simulink model "fast"  (R2019b)
settings: Solver=FixedStepDiscrete  StartTime=0.0  StopTime=25  FixedStep=Ts_proc  RelTol=1e-3
model workspace: external: MAT-File (data not in the file)
values from neighbouring files (symbols this model uses):
  bma = bm + ba    (= 0.0174)    [datasheet.m]
  bp = 0.0024    [datasheet.m]
  CCR_max = 5250    [datasheet.m]
  eta_g = 0.9    [datasheet.m]
  g = 9.81    [datasheet.m]
  J0 = Jm_eq + Jarm + mp*Larm^2    (= 0.0104704670992)    [datasheet.m]
  Jp = Jp_cm + mp*lp^2    (= 0.004290672)    [datasheet.m]
  Ke = 7.68e-3    (= 0.00768)    [datasheet.m]
  Kg = 70    [datasheet.m]
  Kt = 7.68e-3    (= 0.00768)    [datasheet.m]
  Larm = 0.216    [datasheet.m]
  Lm = 0.18*1e-3    (= 0.00018)    [datasheet.m]
  Lp = 0.337    [datasheet.m]
  lp = 0.156    [datasheet.m]
  mp = 0.127    [datasheet.m]
  Rm = 2.6    [datasheet.m]
  Ts_proc = 1e-3    (= 0.001)    [codegen_init.m]
  volt_max = 6    [datasheet.m]
undefined symbols (not defined in the file or in its folder): DiscIntNeverNeededParam, state_pc_init
settings Model: OrderedModelArguments=off  Creator=Simone  LastModifiedBy=Simone
settings OptimizationCC: DefaultParameterBehavior=Inlined  GainParamInheritBuiltInType=on  UseFloatMulNetSlope=on  UseSpecifiedMinMax=on  InlineInvariantSignals=on  PassReuseOutputArgsAs=Individual arguments  ZeroExternalMemoryAtStartup=off  ZeroInternalMemoryAtStartup=off  NoFixptDivByZeroProtection=on  EfficientFloat2IntCast=on  LifeSpan=1  OptimizeBlockOrder=speed  EfficientTunableParamExpr=on
settings DebuggingCC: SignalInfNanChecking=error  ParameterPrecisionLossMsg=error  ParameterTunabilityLossMsg=error
settings HardwareCC: ProdBitPerLong=64  ProdLongLongMode=on  ProdHWDeviceType=Intel->x86-64 (Linux 64)
settings SFSimCC: MATLABDynamicMemAlloc=off
settings RTWCC: SystemTargetFile=ert.tlc  GenCodeOnly=on  PackageGeneratedCodeAndArtifacts=on  TemplateMakefile=ert_default_tmf  GenerateReport=on  Toolchain=GNU gcc/g++ | gmake (64-bit Linux)  BuildConfiguration=Faster Runs  IncludeHyperlinkInReport=on  LaunchReport=on  GenerateTraceInfo=on  GenerateTraceReport=on  GenerateTraceReportSl=on  GenerateTraceReportSf=on  GenerateTraceReportEml=on  CheckMdlBeforeBuild=Error
settings CodeAppCC: ForceParamTrailComments=on  IgnoreCustomStorageClasses=off  OperatorAnnotations=on  SimulinkDataObjDesc=on  SFDataObjDesc=on  MATLABFcnDesc=on  InsertBlockDesc=on  StateflowObjectComments=on  MATLABSourceComments=on  EnableCustomComments=on  ReqsInCode=on
settings ERTTargetCC: TargetLangStandard=C99 (ISO)  UtilityFuncGeneration=Shared location  CombineSignalStateStructs=on  SuppressErrorStatus=on  SupportAbsoluteTime=off  SupportNonFinite=off  SupportComplex=off  InlinedParameterPlacement=NonHierarchical  ERTCustomFileTemplate=example_file_process.tlc

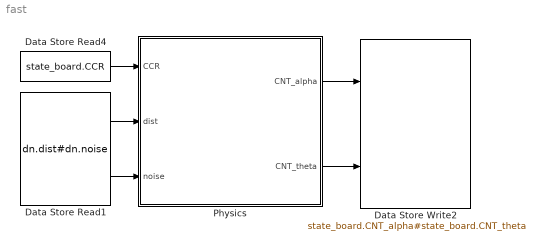
== system fast ==
  Data Store Read1 : DataStoreRead  DataStoreName=dn  DataStoreElements=dn.dist#dn.noise
  Data Store Read4 : DataStoreRead  DataStoreName=state_board  DataStoreElements=state_board.CCR
  Data Store Write2 : DataStoreWrite  DataStoreName=state_board  DataStoreElements=state_board.CNT_alpha#state_board.CNT_theta
  Physics : Subsystem  TreatAsAtomicUnit=on  RTWFcnName=physics  RTWFileName=physics
      settings: RTWSystemCode=Nonreusable function  RTWFcnNameOpts=User specified  RTWFileNameOpts=User specified  FunctionInterfaceSpec=Allow arguments
  wires:
  Data Store Read4/1 -> Physics/1(CCR)
  Physics/1(CNT_alpha) -> Data Store Write2/1
  Physics/2(CNT_theta) -> Data Store Write2/2
  Data Store Read1/1 -> Physics/2(dist)
  Data Store Read1/2 -> Physics/3(noise)

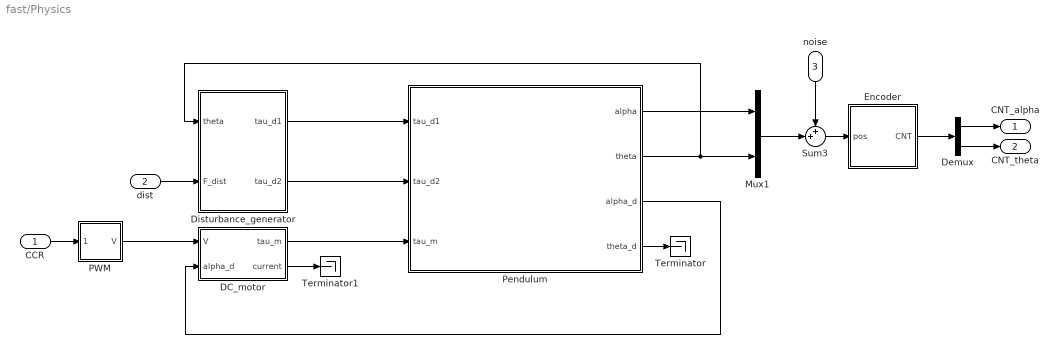
== system fast/Physics ==
  CCR : Inport
  dist : Inport  Port=2
  noise : Inport  Port=3
  DC_motor : Subsystem
  Demux : Demux  Outputs=2
  Disturbance_generator : Subsystem
  Encoder : Subsystem
  Mux1 : Mux  Inputs=2
  PWM : Subsystem
  Pendulum : Subsystem
  Sum3 : Sum  Inputs=++|
  Terminator : Terminator
  Terminator1 : Terminator
  CNT_alpha : Outport
  CNT_theta : Outport  Port=2
  wires:
  Demux/1 -> CNT_alpha/1
  Demux/2 -> CNT_theta/1
  Encoder/1(CNT) -> Demux/1
  Pendulum/4(theta_d) -> Terminator/1
  Mux1/1 -> Sum3/2
  dist/1 -> Disturbance_generator/2(F_dist)
  CCR/1 -> PWM/1(CCR)
  DC_motor/1(tau_m) -> Pendulum/3(tau_m)
  Disturbance_generator/2(tau_d2) -> Pendulum/2(tau_d2)
  Disturbance_generator/1(tau_d1) -> Pendulum/1(tau_d1)
  noise/1 -> Sum3/1
  Sum3/1 -> Encoder/1(pos)
  Pendulum/1(alpha) -> Mux1/1
  Pendulum/2(theta) -> Disturbance_generator/1(theta), Mux1/2
  DC_motor/2(current) -> Terminator1/1
  Pendulum/3(alpha_d) -> DC_motor/2(alpha_d)
  PWM/1(V) -> DC_motor/1(V)

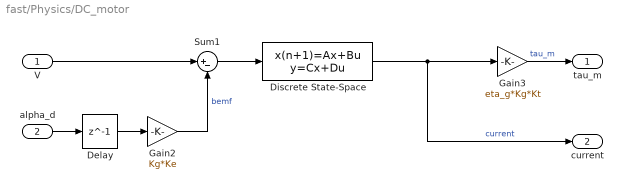
== system fast/Physics/DC_motor ==
  V : Inport
  alpha_d : Inport  Port=2
  Delay : Delay  DelayLength=1  InitialCondition=0
  Discrete State-Space : DiscreteStateSpace  A=-(Rm*Ts_proc - 2*Lm)/(Rm*Ts_proc + 2*Lm)  B=Ts_proc/(2*Lm + Rm*Ts_proc)*(1-(Rm*Ts_proc - 2*Lm)/(Rm*Ts_proc + 2*Lm))  D=Ts_proc/(2*Lm + Rm*Ts_proc)  InitialCondition=single(0)  SampleTime=Ts_proc
  Gain2 : Gain  Gain=Kg*Ke
  Gain3 : Gain  Gain=eta_g*Kg*Kt
  Sum1 : Sum  Inputs=|+-
  tau_m : Outport
  current : Outport  Port=2
  wires:
  Delay/1 -> Gain2/1
  Gain3/1 -> tau_m/1  "tau_m"
  V/1 -> Sum1/1
  alpha_d/1 -> Delay/1
  Discrete State-Space/1 -> current/1, Gain3/1  "current"
  Sum1/1 -> Discrete State-Space/1
  Gain2/1 -> Sum1/2  "bemf"

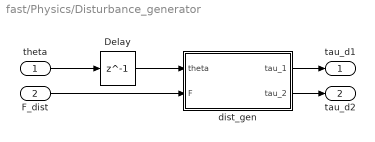
== system fast/Physics/Disturbance_generator ==
  theta : Inport
  F_dist : Inport  Port=2
  Delay : Delay  DelayLength=1  InitialCondition=state_pc_init.theta
  dist_gen : MATLAB Function
  tau_d1 : Outport
  tau_d2 : Outport  Port=2
  wires:
  dist_gen/1(tau_1) -> tau_d1/1
  dist_gen/2(tau_2) -> tau_d2/1
  F_dist/1 -> dist_gen/2(F)
  theta/1 -> Delay/1
  Delay/1 -> dist_gen/1(theta)

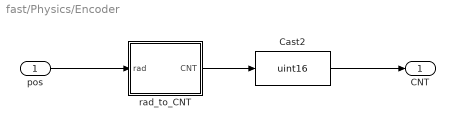
== system fast/Physics/Encoder ==
  pos : Inport
  Cast2 : DataTypeConversion  OutDataTypeStr=uint16
  rad_to_CNT : MATLAB Function
  CNT : Outport
  wires:
  pos/1 -> rad_to_CNT/1(rad)
  Cast2/1 -> CNT/1
  rad_to_CNT/1(CNT) -> Cast2/1

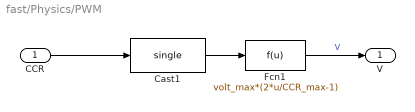
== system fast/Physics/PWM ==
  CCR : Inport
  Cast1 : DataTypeConversion  OutDataTypeStr=single
  Fcn1 : Fcn  Expr=volt_max*(2*u/CCR_max-1)
  V : Outport
  wires:
  CCR/1 -> Cast1/1
  Cast1/1 -> Fcn1/1
  Fcn1/1 -> V/1  "V"

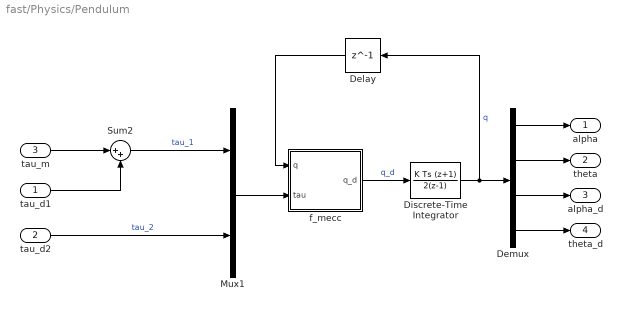
== system fast/Physics/Pendulum ==
  tau_d1 : Inport
  tau_d2 : Inport  Port=2
  tau_m : Inport  Port=3
  Delay : Delay  DelayLength=1  InitialCondition=[state_pc_init.alpha;state_pc_init.theta;0;0]
  Demux : Demux
  Discrete-Time Integrator : DiscreteIntegrator  IntegratorMethod=Integration: Trapezoidal  gainval=single(1.0)  InitialCondition=[state_pc_init.alpha;state_pc_init.theta;0;0]  SampleTime=Ts_proc  ICPrevOutput=DiscIntNeverNeededParam  ICPrevScaledInput=DiscIntNeverNeededParam
  Mux1 : Mux  Inputs=2
  Sum2 : Sum  Inputs=|++
  f_mecc : MATLAB Function  TreatAsAtomicUnit=on
  alpha : Outport
  theta : Outport  Port=2
  alpha_d : Outport  Port=3
  theta_d : Outport  Port=4
  wires:
  Delay/1 -> f_mecc/1(q)
  Demux/2 -> theta/1
  Demux/1 -> alpha/1
  Sum2/1 -> Mux1/1  "tau_1"
  tau_d2/1 -> Mux1/2  "tau_2"
  Discrete-Time Integrator/1 -> Delay/1, Demux/1  "q"
  Mux1/1 -> f_mecc/2(tau)
  f_mecc/1(q_d) -> Discrete-Time Integrator/1  "q_d"
  Demux/3 -> alpha_d/1
  Demux/4 -> theta_d/1
  tau_d1/1 -> Sum2/2
  tau_m/1 -> Sum2/1

== matlab function fast/Physics/Encoder/rad_to_CNT ==
  data: rad input; CNT output; encoder_res parameter
function CNT = rad_to_CNT(rad,encoder_res)

CNT = floor(mod(rad,single(2*pi))/single(2*pi)*encoder_res);

== matlab function fast/Physics/Pendulum/f_mecc ==
  data: q input single; q_d output single; tau input single; mp parameter; J0 parameter; Jp parameter; Larm parameter; lp parameter; g parameter; bma parameter; bp parameter
function q_d = f_mecc(q,tau,mp,J0,Jp,Larm,lp,g,bma,bp)
%#codegen

%    This function was generated by the Symbolic Math Toolbox version 8.4.
%    09-Dec-2019 19:45:31

al_d = q(3);
tau1 = tau(1);
tau2 = tau(2);
th = q(2);
th_d = q(4);
q_d = [al_d;th_d;((Jp.*tau1.*-2.0+Jp.*al_d.*bma.*2.0+Jp.^2.*al_d.*th_d.*sin(th.*2.0).*2.0+Larm.*lp.*mp.*tau2.*cos(th).*2.0-Larm.*bp.*lp.*mp.*th_d.*cos(th).*2.0+Larm.*g.*lp.^2.*mp.^2.*cos(th).*sin(th).*2.0-Jp.*Larm.*lp.*mp.*th_d.^2.*sin(th).*2.0+Jp.*Larm.*al_d.^2.*lp.*mp.*sin(th.*2.0).*cos(th)).*(-1.0./2.0))./(Jp.^2.*sin(th).^2+J0.*Jp-Larm.^2.*lp.^2.*mp.^2.*cos(th).^2);(J0.*tau2.*2.0+Jp.*tau2.*sin(th).^2.*2.0-J0.*bp.*th_d.*2.0+Jp.^2.*al_d.^2.*sin(th.*2.0).*sin(th).^2-Jp.*bp.*th_d.*sin(th).^2.*2.0+J0.*Jp.*al_d.^2.*sin(th.*2.0)+Jp.*g.*lp.*mp.*sin(th).^3.*2.0-Larm.*lp.*mp.*tau1.*cos(th).*2.0+J0.*g.*lp.*mp.*sin(th).*2.0+Larm.*al_d.*bma.*lp.*mp.*cos(th).*2.0-Larm.^2.*lp.^2.*mp.^2.*th_d.^2.*cos(th).*sin(th).*2.0+Jp.*Larm.*al_d.*lp.*mp.*th_d.*sin(th.*2.0).*cos(th).*2.0)./(Jp.^2.*sin(th).^2.*2.0+J0.*Jp.*2.0-Larm.^2.*lp.^2.*mp.^2.*cos(th).^2.*2.0)];

== matlab function fast/Physics/Disturbance_generator/dist_gen ==
  data: theta input; F input; tau_1 output single; tau_2 output single; Larm parameter; Lp parameter
function [tau_1,tau_2] = dist_gen(theta,F,Larm,Lp)

tau_1 = F*Larm;
tau_2 = F*cos(theta)*Lp;
